simulink model "navigator"  (R2013b)
settings: Solver=FixedStepDiscrete  StartTime=0.0  StopTime=inf  FixedStep=0.2  RelTol=1e-3
undefined symbols (not defined in the file): Earth, WGS84
libraries: aerolibtransform2 x2, simulink_extras x1
settings Model: Creator=Matteo  LastModifiedBy=Gianluca Rossetti
settings OptimizationCC: OptimizeModelRefInitCode=on  LifeSpan=Inf
settings HardwareCC: ProdBitPerInt=16  ProdBitPerPointer=8  ProdIntDivRoundTo=Zero  ProdEndianess=LittleEndian  ProdWordSize=8  ProdHWDeviceType=Atmel->AVR
settings RTWCC: SystemTargetFile=ert.tlc  GenCodeOnly=on  TemplateMakefile=ert_default_tmf  Description=Embedded Coder  ProcessScript=ert_make_rtw_hook  BuildConfiguration=Faster Runs  TargetLang=C++  CheckMdlBeforeBuild=Warning
settings CodeAppCC: IgnoreCustomStorageClasses=off
settings ERTTargetCC: CodeReplacementLibrary=ANSI_C  GenerateSampleERTMain=on  ERTCustomFileTemplate=example_file_process.tlc

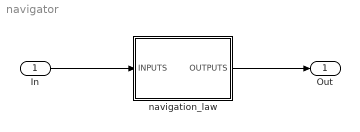
== system navigator ==
  In : Inport  OutDataTypeStr=single  PortDimensions=21
  navigation_law : Subsystem
  Out : Outport  OutDataTypeStr=single  PortDimensions=15
  wires:
  In/1 -> navigation_law/1(INPUTS)
  navigation_law/1(OUTPUTS) -> Out/1

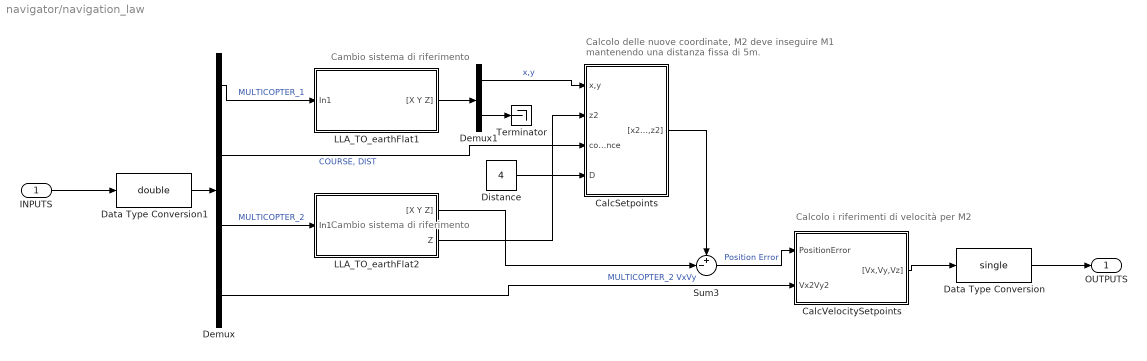
== system navigator/navigation_law ==
  note: Cambio sistema di riferimento
  note: Cambio sistema di riferimento
  note: Calcolo delle nuove coordinate, M2 deve
      | inseguire M1 mantenendo una distanza fissa di 5m.
  note: Calcolo i riferimenti di velocità per M2
  INPUTS : Inport  PortDimensions=14
  CalcSetpoints : Subsystem
  CalcVelocitySetpoints : Subsystem
  Data Type Conversion : DataTypeConversion  OutDataTypeStr=single
  Data Type Conversion1 : DataTypeConversion  OutDataTypeStr=double
  Demux : Demux  Outputs=[5 2 5 2]
  Demux1 : Demux  Outputs=[2 1]
  Distance : Constant  Value=4
  LLA_TO_earthFlat1 : Subsystem
  LLA_TO_earthFlat2 : Subsystem
  Sum3 : Sum  Inputs=+-|
  Terminator : Terminator
  OUTPUTS : Outport  PortDimensions=3
  wires:
  Demux/3 -> LLA_TO_earthFlat2/1(In1)  "MULTICOPTER_2"
  INPUTS/1 -> Data Type Conversion1/1
  Data Type Conversion1/1 -> Demux/1
  Demux/1 -> LLA_TO_earthFlat1/1(In1)  "MULTICOPTER_1"
  Demux/2 -> CalcSetpoints/3("course, distance")  "COURSE, DIST"
  LLA_TO_earthFlat1/1("[X Y Z]") -> Demux1/1
  Demux1/1 -> CalcSetpoints/1(x,y)  "x,y"
  LLA_TO_earthFlat2/2(Z) -> CalcSetpoints/2(z2)
  Distance/1 -> CalcSetpoints/4(D)
  Sum3/1 -> CalcVelocitySetpoints/1(PositionError)  "Position Error"
  LLA_TO_earthFlat2/1("[X Y Z]") -> Sum3/2
  CalcSetpoints/1("[x2,y2,z2]") -> Sum3/1
  CalcVelocitySetpoints/1("[Vx,Vy,Vz]") -> Data Type Conversion/1
  Data Type Conversion/1 -> OUTPUTS/1
  Demux1/2 -> Terminator/1
  Demux/4 -> CalcVelocitySetpoints/2(Vx2Vy2)  "MULTICOPTER_2 VxVy"

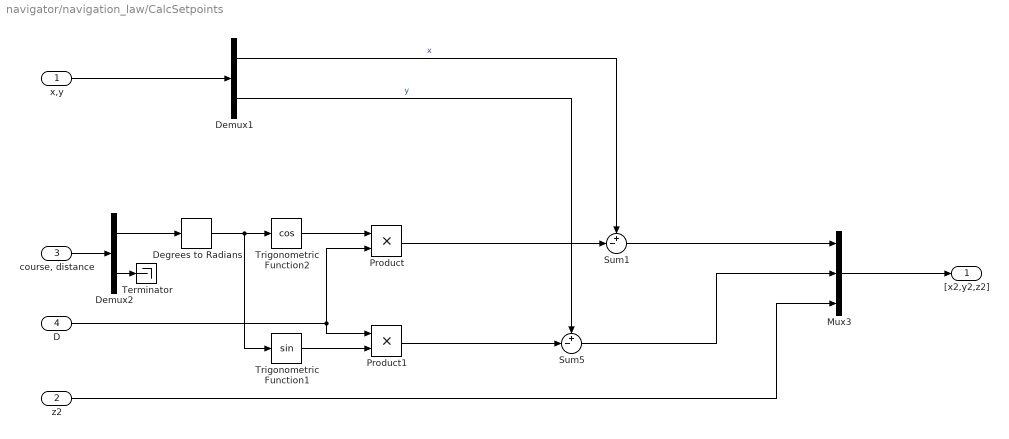
== system navigator/navigation_law/CalcSetpoints ==
  x,y : Inport
  z2 : Inport  Port=2
  "course, distance" : Inport  Port=3
  D : Inport  Port=4
  Degrees to Radians : simulink_extras/Transformations/Degrees to Radians
  Demux1 : Demux  Outputs=[1 1]
  Demux2 : Demux  Outputs=[1 1]
  Mux3 : Mux  Inputs=[1 1 1]
  Product : Product
  Product1 : Product
  Sum1 : Sum  Inputs=+-|
  Sum5 : Sum  Inputs=+-|
  Terminator : Terminator
  Trigonometric Function1 : Trigonometry
  Trigonometric Function2 : Trigonometry  Operator=cos
  "[x2,y2,z2]" : Outport
  wires:
  Mux3/1 -> "[x2,y2,z2]"/1
  Product1/1 -> Sum5/2
  "course, distance"/1 -> Demux2/1
  Demux1/2 -> Sum5/1  "y"
  Product/1 -> Sum1/2
  D/1 -> Product1/1, Product/2
  x,y/1 -> Demux1/1
  Degrees to Radians/1 -> Trigonometric Function1/1, Trigonometric Function2/1
  Trigonometric Function2/1 -> Product/1
  Trigonometric Function1/1 -> Product1/2
  Demux1/1 -> Sum1/1  "x"
  Sum1/1 -> Mux3/1
  Sum5/1 -> Mux3/2
  z2/1 -> Mux3/3
  Demux2/1 -> Degrees to Radians/1
  Demux2/2 -> Terminator/1

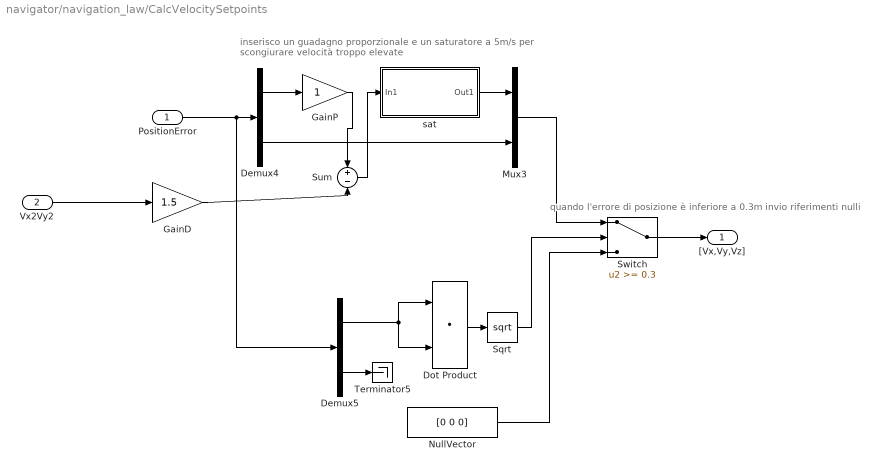
== system navigator/navigation_law/CalcVelocitySetpoints ==
  note: inserisco un guadagno proporzionale e un saturatore a 5m/s
      | per scongiurare velocità troppo elevate
  note: quando l'errore di posizione è inferiore a 0.3m invio riferimenti nulli
  PositionError : Inport
  Vx2Vy2 : Inport  Port=2
  Demux4 : Demux  Outputs=[2 1]
  Demux5 : Demux  Outputs=[2 1]
  Dot Product : DotProduct  InputSameDT=on  OutDataTypeStr=Inherit: Inherit via internal rule
  GainD : Gain  Gain=1.5
  GainP : Gain
  Mux3 : Mux  Inputs=[2 1]
  NullVector : Constant  Value=[0 0 0]
  Sqrt : Sqrt  SaturateOnIntegerOverflow=on
  Sum : Sum  Inputs=+-
  Switch : Switch  Threshold=0.3
  Terminator5 : Terminator
  "sat " : Subsystem  mask{k_sat=5}
      mask prompts: k_sat "Saturatore"
  "[Vx,Vy,Vz]" : Outport
  wires:
  Switch/1 -> "[Vx,Vy,Vz]"/1
  NullVector/1 -> Switch/3
  Mux3/1 -> Switch/1
  Sqrt/1 -> Switch/2
  Demux5/2 -> Terminator5/1
  Dot Product/1 -> Sqrt/1
  Demux5/1 -> Dot Product/2, Dot Product/1
  Demux4/2 -> Mux3/2
  "sat "/1(Out1) -> Mux3/1
  Demux4/1 -> GainP/1
  PositionError/1 -> Demux4/1, Demux5/1
  GainP/1 -> Sum/1
  Vx2Vy2/1 -> GainD/1
  GainD/1 -> Sum/2
  Sum/1 -> "sat "/1(In1)

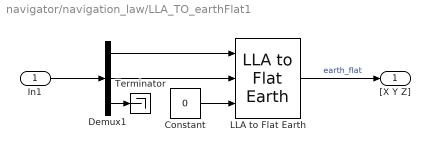
== system navigator/navigation_law/LLA_TO_earthFlat1 ==
  In1 : Inport
  Constant : Constant  Value=0  OutDataTypeStr=single
  Demux1 : Demux  Outputs=[2 1 2]
  LLA to Flat Earth : aerolibtransform2/LLA to Flat Earth  units=Metric (MKS)  ptype=Earth (WGS84)  F=1/298.257223563  R=6378137  LL0="[44.201892800000003  12.062565800000000]"  psi=0
  Terminator : Terminator
  "[X Y Z]" : Outport
  wires:
  Demux1/3 -> Terminator/1
  In1/1 -> Demux1/1
  Demux1/2 -> LLA to Flat Earth/2
  LLA to Flat Earth/1 -> "[X Y Z]"/1  "earth_flat"
  Demux1/1 -> LLA to Flat Earth/1
  Constant/1 -> LLA to Flat Earth/3

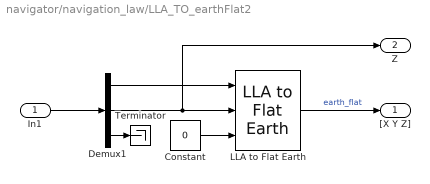
== system navigator/navigation_law/LLA_TO_earthFlat2 ==
  In1 : Inport
  Constant : Constant  Value=0  OutDataTypeStr=single
  Demux1 : Demux  Outputs=[2 1 2]
  LLA to Flat Earth : aerolibtransform2/LLA to Flat Earth  units=Metric (MKS)  ptype=Earth (WGS84)  F=1/298.257223563  R=6378137  LL0="[44.201892800000003  12.062565800000000]"  psi=0
  Terminator : Terminator
  "[X Y Z]" : Outport
  Z : Outport  Port=2
  wires:
  Constant/1 -> LLA to Flat Earth/3
  Demux1/1 -> LLA to Flat Earth/1
  LLA to Flat Earth/1 -> "[X Y Z]"/1  "earth_flat"
  Demux1/2 -> Z/1, LLA to Flat Earth/2
  In1/1 -> Demux1/1
  Demux1/3 -> Terminator/1

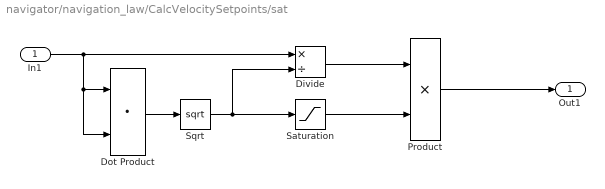
== system navigator/navigation_law/CalcVelocitySetpoints/sat  ==
  In1 : Inport
  Divide : Product  Inputs=*/
  Dot Product : DotProduct  InputSameDT=on  OutDataTypeStr=Inherit: Inherit via internal rule
  Product : Product
  Saturation : Saturate  UpperLimit=k_sat  LowerLimit=0
  Sqrt : Sqrt  SaturateOnIntegerOverflow=on
  Out1 : Outport
  wires:
  Saturation/1 -> Product/2
  Dot Product/1 -> Sqrt/1
  In1/1 -> Dot Product/2, Dot Product/1, Divide/1
  Sqrt/1 -> Saturation/1, Divide/2
  Product/1 -> Out1/1
  Divide/1 -> Product/1
